simulink model "task_2_3"  (R2024a)
settings: Solver=VariableStepAuto  StartTime=0.0  StopTime=30.0  RelTol=1e-3
settings Model: Creator=alexe  LastModifiedBy=alexe

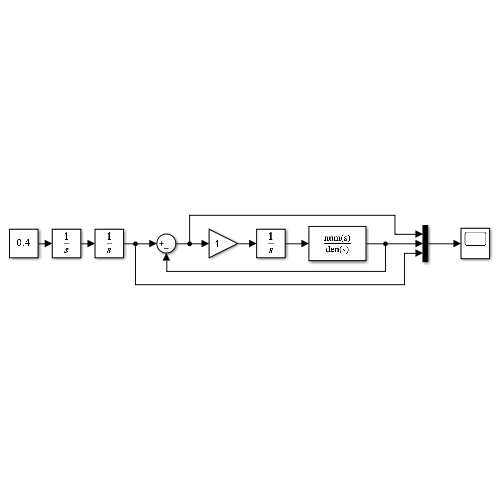
[thumbnail: Simulink's stored preview of the top-level diagram]
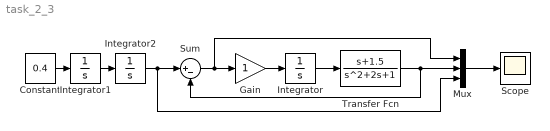
== system task_2_3 ==
  Constant : Constant  Value=0.4
  Gain : Gain
  Integrator : Integrator
  Integrator1 : Integrator
  Integrator2 : Integrator
  Mux : Mux  Inputs=3
  Scope : Scope
  Sum : Sum  Inputs=|+-
  Transfer Fcn : TransferFcn  Numerator=[1 1.5]
  wires:
  Integrator2/1 -> Mux/3, Sum/1
  Sum/1 -> Gain/1, Mux/1
  Integrator/1 -> Transfer Fcn/1
  Transfer Fcn/1 -> Mux/2, Sum/2
  Mux/1 -> Scope/1
  Gain/1 -> Integrator/1
  Constant/1 -> Integrator1/1
  Integrator1/1 -> Integrator2/1
